simulink library "CTRL_SPECCTRL_FB"  (R2024b)
settings: Solver=VariableStepAuto  StartTime=0.0  StopTime=10.0  RelTol=1e-3
libraries: CTRL_SPECCTRL_FB_STRAT1 x1, CTRL_SPECCTRL_FB_STRAT2 x1, CTRL_SPECCTRL_FB_STRAT3 x1
settings Model: Creator=blatak  LastModifiedBy=blatak

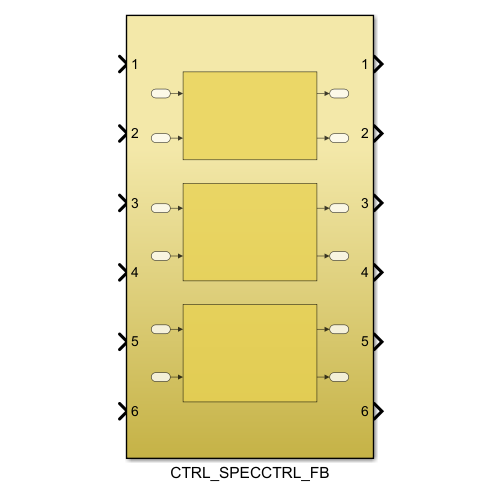
[thumbnail: Simulink's stored preview of the top-level diagram]
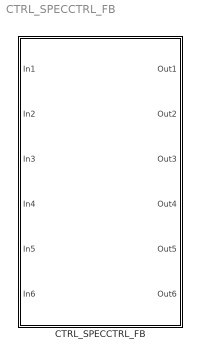
== system CTRL_SPECCTRL_FB ==
  CTRL_SPECCTRL_FB : Subsystem

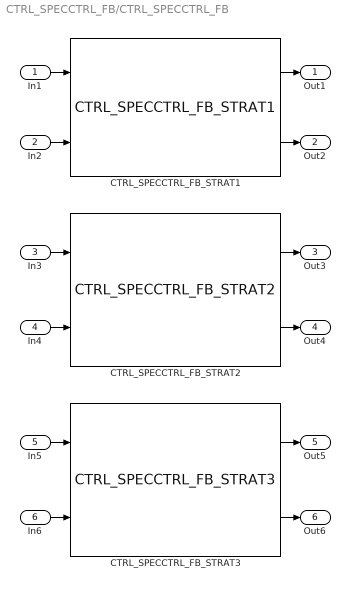
== system CTRL_SPECCTRL_FB/CTRL_SPECCTRL_FB ==
  In1 : Inport
  In2 : Inport  Port=2
  In3 : Inport  Port=3
  In4 : Inport  Port=4
  In5 : Inport  Port=5
  In6 : Inport  Port=6
  CTRL_SPECCTRL_FB_STRAT1 : CTRL_SPECCTRL_FB_STRAT1/CTRL_SPECCTRL_FB_STRAT1  SystemSampleTime=-1  VariantActivationTime=update diagram  AllowFlexibleInterface=on  Latency=0  AutoFrameSizeCalculation=off
  CTRL_SPECCTRL_FB_STRAT2 : CTRL_SPECCTRL_FB_STRAT2/CTRL_SPECCTRL_FB_STRAT2  SystemSampleTime=-1  VariantActivationTime=update diagram  AllowFlexibleInterface=on  Latency=0  AutoFrameSizeCalculation=off
  CTRL_SPECCTRL_FB_STRAT3 : CTRL_SPECCTRL_FB_STRAT3/CTRL_SPECCTRL_FB_STRAT3  SystemSampleTime=-1  VariantActivationTime=update diagram  AllowFlexibleInterface=on  Latency=0  AutoFrameSizeCalculation=off
  Out1 : Outport
  Out2 : Outport  Port=2
  Out3 : Outport  Port=3
  Out4 : Outport  Port=4
  Out5 : Outport  Port=5
  Out6 : Outport  Port=6
  wires:
  CTRL_SPECCTRL_FB_STRAT1/1 -> Out1/1
  CTRL_SPECCTRL_FB_STRAT3/2 -> Out6/1
  CTRL_SPECCTRL_FB_STRAT3/1 -> Out5/1
  In3/1 -> CTRL_SPECCTRL_FB_STRAT2/1
  In4/1 -> CTRL_SPECCTRL_FB_STRAT2/2
  In6/1 -> CTRL_SPECCTRL_FB_STRAT3/2
  CTRL_SPECCTRL_FB_STRAT2/1 -> Out3/1
  CTRL_SPECCTRL_FB_STRAT2/2 -> Out4/1
  In1/1 -> CTRL_SPECCTRL_FB_STRAT1/1
  CTRL_SPECCTRL_FB_STRAT1/2 -> Out2/1
  In5/1 -> CTRL_SPECCTRL_FB_STRAT3/1
  In2/1 -> CTRL_SPECCTRL_FB_STRAT1/2
